simulink model "main_sim"  (R2021b)
settings: Solver=ode1  StartTime=0.0  StopTime=10000000000000000  FixedStep=1  RelTol=1e-3
settings Model: Creator=alexs  LastModifiedBy=alexs

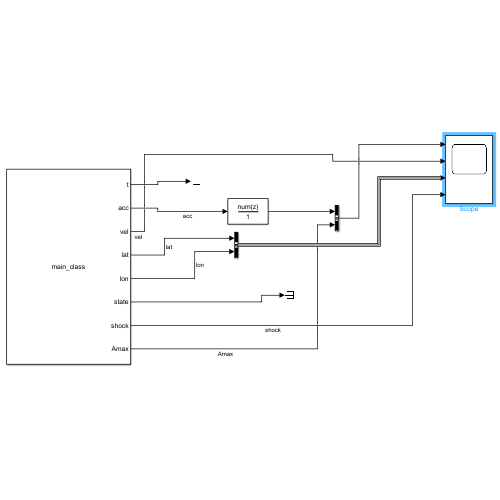
[thumbnail: Simulink's stored preview of the top-level diagram]
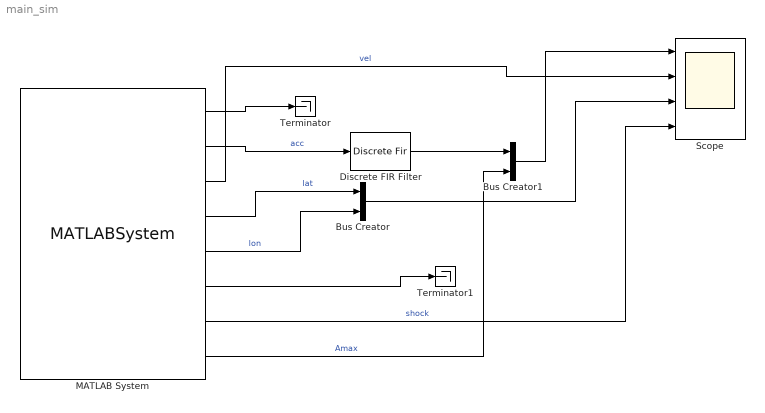
== system main_sim ==
  Bus Creator : BusCreator  Inputs=2
  Bus Creator1 : BusCreator  Inputs=2
  Discrete FIR Filter : DiscreteFir  Coefficients="[0.183297562620086   0.202106574665581   0.208660314019862   0.202106574665581   0.183297562620086]"
  MATLAB System : MATLABSystem  System=main_class  SimulateUsing=Interpreted execution
      mask Type: main_class
      mask Display:
      | disp('main_class');
      | port_label('output',1,'t');
      | port_label('output',2,'acc');
      | port_label('output',3,'vel');
      | port_label('output',4,'lat');
      | port_label('output',5,'lon');
      | port_label('output',6,'state');
      | port_label('output',7,'shock');
      | port_label('output',8,'Amax');
  Scope : Scope  NumInputPorts=4
  Terminator : Terminator
  Terminator1 : Terminator
  wires:
  MATLAB System/2 -> Discrete FIR Filter/1  "acc"
  MATLAB System/3 -> Scope/2  "vel"
  MATLAB System/4 -> Bus Creator/1  "lat"
  MATLAB System/5 -> Bus Creator/2  "lon"
  Bus Creator/1 -> Scope/3
  MATLAB System/1 -> Terminator/1
  MATLAB System/6 -> Terminator1/1
  MATLAB System/8 -> Bus Creator1/2  "Amax"
  Discrete FIR Filter/1 -> Bus Creator1/1
  Bus Creator1/1 -> Scope/1
  MATLAB System/7 -> Scope/4  "shock"
